simulink model "hw7_systtem"  (R2015a)
settings: Solver=ode45  StartTime=0.0  StopTime=10.0  RelTol=1e-3
settings Model: Creator=lbremer  LastModifiedBy=lbremer

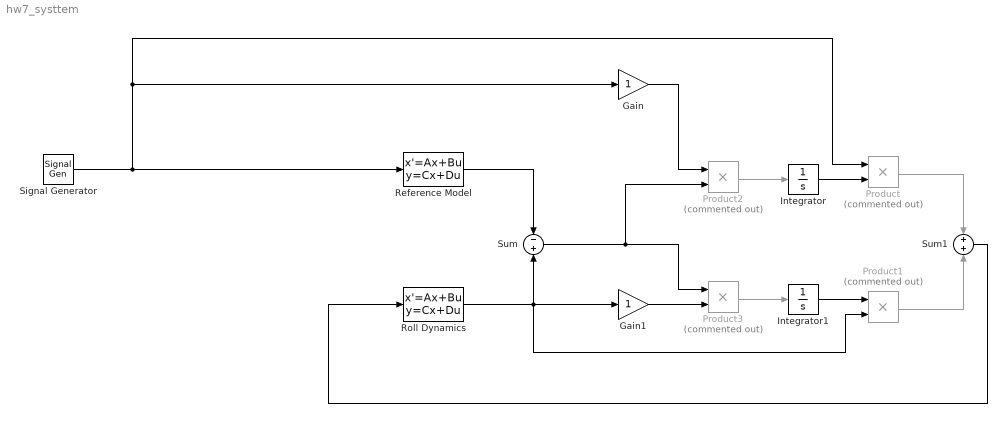
== system hw7_systtem ==
  Gain : Gain
  Gain1 : Gain
  Integrator : Integrator
  Integrator1 : Integrator
  Product{,1..3} (4 alike) : Product  Commented=on
  Reference Model : StateSpace  X0=0
  Roll Dynamics : StateSpace  X0=0
  Signal Generator : SignalGenerator  Units=rad/sec
  Sum : Sum  Inputs=-|+
  Sum1 : Sum  Inputs=+|+
  wires:
  Reference Model/1 -> Sum/1
  Gain/1 -> Product2/1
  Sum/1 -> Product3/1, Product2/2
  Gain1/1 -> Product3/2
  Product2/1 -> Integrator/1
  Product3/1 -> Integrator1/1
  Integrator/1 -> Product/2
  Signal Generator/1 -> Product/1, Gain/1, Reference Model/1
  Integrator1/1 -> Product1/1
  Roll Dynamics/1 -> Gain1/1, Product1/2, Sum/2
  Product/1 -> Sum1/1
  Product1/1 -> Sum1/2
  Sum1/1 -> Roll Dynamics/1
